simulink model "T4_ongrid_updatesolar"  (R2022b)
settings: Solver=FixedStepAuto  StartTime=0.0  StopTime=24  FixedStep=0.01  RelTol=1e-3
undefined symbols (not defined in the file): High, Low, Ts
libraries: fl_lib x142, nesl_utility x59, simulink x15, ee_lib x8, batteryecm_lib x1
(part 2 of 3)

== system T4_ongrid_updatesolar/Household8 ==
  Current Sensor : fl_lib/Electrical/Electrical Sensors/Current Sensor
  PS Divide : fl_lib/Physical Signals/Functions/PS Divide
  PS Product : fl_lib/Physical Signals/Functions/PS Product
  PS-Simulink Converter : nesl_utility/PS-Simulink Converter  PhysicalDomain=network_engine_domain  SubClassName=ps_output  LeftPortType=input  RightPortType=output  PseudoPeriodic=off  Frequencies=[]  VectorFormat=inherit  Unit=inherit  AffineConversion=off
  PS-Simulink Converter1 : nesl_utility/PS-Simulink Converter  PhysicalDomain=network_engine_domain  SubClassName=ps_output  LeftPortType=input  RightPortType=output  PseudoPeriodic=off  Frequencies=[]  VectorFormat=inherit  Unit=inherit  AffineConversion=off
  Product : Product
  "Residential power " : simulink/Sources/Repeating Sequence Interpolated  OutValues=[2.8 2.5 2 2 2.2 2.5 2.8 3.4 3.6 3.8 4 4 4 4 4 4 4 4 4 4 3.8 3.5 3.2 3]*1000  TimeValues=[0 1 2 3 4 5 6 7 8 9 10 11 12 13 14 15 16 17 18 19 20 21 22 23]  LookUpMeth=Interpolation-Use End Values  tsamp=0.01  OutMin=[]  OutMax=[]  OutDataTypeStr=double  OutputDataTypeScalingMode=double  OutDataType=fixdt(0,8)  OutScaling=2^-10
  Simscape Bus1 : SimscapeBus  HierarchyStrings=High;Low
  Simulink-PS Converter1 : nesl_utility/Simulink-PS Converter  PhysicalDomain=network_engine_domain  SubClassName=ps_input  LeftPortType=input  RightPortType=output  PseudoPeriodic=off  Frequencies=[]  NoiseDistribution=none  NoiseParameters=[]  Unit=V*A  AffineConversion=off  FilteringAndDerivatives=provide  SimscapeFilterOrder=1  InputFilterTimeConstant=0.001  UdotUserProvided=0
  Terminator : Terminator
  Variable Resistor : fl_lib/Electrical/Electrical Elements/Variable Resistor  Rmin=0 Ohm  i_specify=off  i_priority=None  i=0 A  i_nominal_specify=off  i_nominal_unit=A  i_nominal_value=1  v_specify=off  v_priority=None  v=0 V  v_nominal_specify=off  v_nominal_unit=V  v_nominal_value=1
  Vnom : fl_lib/Physical Signals/Sources/PS Constant  constant=48 V
  Voltage Sensor : fl_lib/Electrical/Electrical Sensors/Voltage Sensor
  IndustrialOut : PMIOPort  Side=Right
  wires:
  Product/1 -> Terminator/1  "power"
  PS-Simulink Converter1/1 -> Product/1  "current"
  PS-Simulink Converter/1 -> Product/2  "voltage"
  "Residential power "/1 -> Simulink-PS Converter1/1  "electrical"
  connections:
  Current Sensor/RConn1 -- PS-Simulink Converter1/LConn1
  Current Sensor/LConn1 -- Simscape Bus1/LConn1
  Voltage Sensor/RConn1 -- PS-Simulink Converter/LConn1
  Current Sensor/RConn2 -- Variable Resistor/LConn2 -- Voltage Sensor/LConn1
  IndustrialOut/RConn1 -- Simscape Bus1/RConn1
  Voltage Sensor/RConn2 -- Simscape Bus1/LConn2 -- Variable Resistor/RConn1
  Vnom/RConn1 -- PS Product/LConn2 -- PS Product/LConn1
  PS Divide/LConn2 -- Simulink-PS Converter1/RConn1
  Variable Resistor/LConn1 -- PS Divide/RConn1
  PS Divide/LConn1 -- PS Product/RConn1

== system T4_ongrid_updatesolar/Household9 ==
  Current Sensor : fl_lib/Electrical/Electrical Sensors/Current Sensor
  PS Divide : fl_lib/Physical Signals/Functions/PS Divide
  PS Product : fl_lib/Physical Signals/Functions/PS Product
  PS-Simulink Converter : nesl_utility/PS-Simulink Converter  PhysicalDomain=network_engine_domain  SubClassName=ps_output  LeftPortType=input  RightPortType=output  PseudoPeriodic=off  Frequencies=[]  VectorFormat=inherit  Unit=inherit  AffineConversion=off
  PS-Simulink Converter1 : nesl_utility/PS-Simulink Converter  PhysicalDomain=network_engine_domain  SubClassName=ps_output  LeftPortType=input  RightPortType=output  PseudoPeriodic=off  Frequencies=[]  VectorFormat=inherit  Unit=inherit  AffineConversion=off
  Product : Product
  "Residential power " : simulink/Sources/Repeating Sequence Interpolated  OutValues=[2.8 2.5 2 2 2.2 2.5 2.8 3.4 3.6 3.8 4 4 4 4 4 4 4 4 4 4 3.8 3.5 3.2 3]*1000  TimeValues=[0 1 2 3 4 5 6 7 8 9 10 11 12 13 14 15 16 17 18 19 20 21 22 23]  LookUpMeth=Interpolation-Use End Values  tsamp=0.01  OutMin=[]  OutMax=[]  OutDataTypeStr=double  OutputDataTypeScalingMode=double  OutDataType=fixdt(0,8)  OutScaling=2^-10
  Simscape Bus1 : SimscapeBus  HierarchyStrings=High;Low
  Simulink-PS Converter1 : nesl_utility/Simulink-PS Converter  PhysicalDomain=network_engine_domain  SubClassName=ps_input  LeftPortType=input  RightPortType=output  PseudoPeriodic=off  Frequencies=[]  NoiseDistribution=none  NoiseParameters=[]  Unit=V*A  AffineConversion=off  FilteringAndDerivatives=provide  SimscapeFilterOrder=1  InputFilterTimeConstant=0.001  UdotUserProvided=0
  Terminator : Terminator
  Variable Resistor : fl_lib/Electrical/Electrical Elements/Variable Resistor  Rmin=0 Ohm  i_specify=off  i_priority=None  i=0 A  i_nominal_specify=off  i_nominal_unit=A  i_nominal_value=1  v_specify=off  v_priority=None  v=0 V  v_nominal_specify=off  v_nominal_unit=V  v_nominal_value=1
  Vnom : fl_lib/Physical Signals/Sources/PS Constant  constant=48 V
  Voltage Sensor : fl_lib/Electrical/Electrical Sensors/Voltage Sensor
  IndustrialOut : PMIOPort  Side=Right
  wires:
  Product/1 -> Terminator/1  "power"
  PS-Simulink Converter1/1 -> Product/1  "current"
  PS-Simulink Converter/1 -> Product/2  "voltage"
  "Residential power "/1 -> Simulink-PS Converter1/1  "electrical"
  connections:
  Current Sensor/RConn1 -- PS-Simulink Converter1/LConn1
  Current Sensor/LConn1 -- Simscape Bus1/LConn1
  Voltage Sensor/RConn1 -- PS-Simulink Converter/LConn1
  Current Sensor/RConn2 -- Variable Resistor/LConn2 -- Voltage Sensor/LConn1
  IndustrialOut/RConn1 -- Simscape Bus1/RConn1
  Voltage Sensor/RConn2 -- Simscape Bus1/LConn2 -- Variable Resistor/RConn1
  Vnom/RConn1 -- PS Product/LConn2 -- PS Product/LConn1
  PS Divide/LConn2 -- Simulink-PS Converter1/RConn1
  Variable Resistor/LConn1 -- PS Divide/RConn1
  PS Divide/LConn1 -- PS Product/RConn1

== system T4_ongrid_updatesolar/Line1 ==
  Resistor : fl_lib/Electrical/Electrical Elements/Resistor  R=rho*l/A Ohm  i_specify=off  i_priority=None  i=0 A  i_nominal_specify=off  i_nominal_unit=A  i_nominal_value=1  v_specify=off  v_priority=None  v=0 V  v_nominal_specify=off  v_nominal_unit=V  v_nominal_value=1
  Resistor1 : fl_lib/Electrical/Electrical Elements/Resistor  R=rho*l/A Ohm  i_specify=off  i_priority=None  i=0 A  i_nominal_specify=off  i_nominal_unit=A  i_nominal_value=1  v_specify=off  v_priority=None  v=0 V  v_nominal_specify=off  v_nominal_unit=V  v_nominal_value=1
  Simscape Bus2 : SimscapeBus  HierarchyStrings=High;Low
  Simscape Bus3 : SimscapeBus  HierarchyStrings=High;Low
  In : PMIOPort  Side=Left
  Out : PMIOPort  Port=2  Side=Right
  connections:
  Simscape Bus2/LConn1 -- Resistor/LConn1
  Simscape Bus3/LConn2 -- Resistor1/RConn1
  Simscape Bus2/RConn1 -- In/RConn1
  Simscape Bus3/LConn1 -- Resistor/RConn1
  Resistor1/LConn1 -- Simscape Bus2/LConn2
  Simscape Bus3/RConn1 -- Out/RConn1

== system T4_ongrid_updatesolar/Line10 ==
  Resistor : fl_lib/Electrical/Electrical Elements/Resistor  R=rho*l/A Ohm  i_specify=off  i_priority=None  i=0 A  i_nominal_specify=off  i_nominal_unit=A  i_nominal_value=1  v_specify=off  v_priority=None  v=0 V  v_nominal_specify=off  v_nominal_unit=V  v_nominal_value=1
  Resistor1 : fl_lib/Electrical/Electrical Elements/Resistor  R=rho*l/A Ohm  i_specify=off  i_priority=None  i=0 A  i_nominal_specify=off  i_nominal_unit=A  i_nominal_value=1  v_specify=off  v_priority=None  v=0 V  v_nominal_specify=off  v_nominal_unit=V  v_nominal_value=1
  Simscape Bus2 : SimscapeBus  HierarchyStrings=High;Low
  Simscape Bus3 : SimscapeBus  HierarchyStrings=High;Low
  In : PMIOPort  Side=Left
  Out : PMIOPort  Port=2  Side=Right
  connections:
  Simscape Bus2/LConn1 -- Resistor/LConn1
  Simscape Bus3/LConn2 -- Resistor1/RConn1
  Simscape Bus2/RConn1 -- In/RConn1
  Simscape Bus3/LConn1 -- Resistor/RConn1
  Resistor1/LConn1 -- Simscape Bus2/LConn2
  Simscape Bus3/RConn1 -- Out/RConn1

== system T4_ongrid_updatesolar/Line11 ==
  Resistor : fl_lib/Electrical/Electrical Elements/Resistor  R=rho*l/A Ohm  i_specify=off  i_priority=None  i=0 A  i_nominal_specify=off  i_nominal_unit=A  i_nominal_value=1  v_specify=off  v_priority=None  v=0 V  v_nominal_specify=off  v_nominal_unit=V  v_nominal_value=1
  Resistor1 : fl_lib/Electrical/Electrical Elements/Resistor  R=rho*l/A Ohm  i_specify=off  i_priority=None  i=0 A  i_nominal_specify=off  i_nominal_unit=A  i_nominal_value=1  v_specify=off  v_priority=None  v=0 V  v_nominal_specify=off  v_nominal_unit=V  v_nominal_value=1
  Simscape Bus2 : SimscapeBus  HierarchyStrings=High;Low
  Simscape Bus3 : SimscapeBus  HierarchyStrings=High;Low
  In : PMIOPort  Side=Left
  Out : PMIOPort  Port=2  Side=Right
  connections:
  Simscape Bus3/RConn1 -- Out/RConn1
  Resistor1/LConn1 -- Simscape Bus2/LConn2
  Simscape Bus3/LConn1 -- Resistor/RConn1
  Simscape Bus2/RConn1 -- In/RConn1
  Simscape Bus3/LConn2 -- Resistor1/RConn1
  Simscape Bus2/LConn1 -- Resistor/LConn1

== system T4_ongrid_updatesolar/Line12 ==
  Resistor : fl_lib/Electrical/Electrical Elements/Resistor  R=rho*l/A Ohm  i_specify=off  i_priority=None  i=0 A  i_nominal_specify=off  i_nominal_unit=A  i_nominal_value=1  v_specify=off  v_priority=None  v=0 V  v_nominal_specify=off  v_nominal_unit=V  v_nominal_value=1
  Resistor1 : fl_lib/Electrical/Electrical Elements/Resistor  R=rho*l/A Ohm  i_specify=off  i_priority=None  i=0 A  i_nominal_specify=off  i_nominal_unit=A  i_nominal_value=1  v_specify=off  v_priority=None  v=0 V  v_nominal_specify=off  v_nominal_unit=V  v_nominal_value=1
  Simscape Bus2 : SimscapeBus  HierarchyStrings=High;Low
  Simscape Bus3 : SimscapeBus  HierarchyStrings=High;Low
  In : PMIOPort  Side=Left
  Out : PMIOPort  Port=2  Side=Right
  connections:
  Simscape Bus3/RConn1 -- Out/RConn1
  Resistor1/LConn1 -- Simscape Bus2/LConn2
  Simscape Bus3/LConn1 -- Resistor/RConn1
  Simscape Bus2/RConn1 -- In/RConn1
  Simscape Bus3/LConn2 -- Resistor1/RConn1
  Simscape Bus2/LConn1 -- Resistor/LConn1

== system T4_ongrid_updatesolar/Line13 ==
  Resistor : fl_lib/Electrical/Electrical Elements/Resistor  R=rho*l/A Ohm  i_specify=off  i_priority=None  i=0 A  i_nominal_specify=off  i_nominal_unit=A  i_nominal_value=1  v_specify=off  v_priority=None  v=0 V  v_nominal_specify=off  v_nominal_unit=V  v_nominal_value=1
  Resistor1 : fl_lib/Electrical/Electrical Elements/Resistor  R=rho*l/A Ohm  i_specify=off  i_priority=None  i=0 A  i_nominal_specify=off  i_nominal_unit=A  i_nominal_value=1  v_specify=off  v_priority=None  v=0 V  v_nominal_specify=off  v_nominal_unit=V  v_nominal_value=1
  Simscape Bus2 : SimscapeBus  HierarchyStrings=High;Low
  Simscape Bus3 : SimscapeBus  HierarchyStrings=High;Low
  In : PMIOPort  Side=Left
  Out : PMIOPort  Port=2  Side=Right
  connections:
  Simscape Bus2/LConn1 -- Resistor/LConn1
  Simscape Bus3/LConn2 -- Resistor1/RConn1
  Simscape Bus2/RConn1 -- In/RConn1
  Simscape Bus3/LConn1 -- Resistor/RConn1
  Resistor1/LConn1 -- Simscape Bus2/LConn2
  Simscape Bus3/RConn1 -- Out/RConn1

== system T4_ongrid_updatesolar/Line14 ==
  Resistor : fl_lib/Electrical/Electrical Elements/Resistor  R=rho*l/A Ohm  i_specify=off  i_priority=None  i=0 A  i_nominal_specify=off  i_nominal_unit=A  i_nominal_value=1  v_specify=off  v_priority=None  v=0 V  v_nominal_specify=off  v_nominal_unit=V  v_nominal_value=1
  Resistor1 : fl_lib/Electrical/Electrical Elements/Resistor  R=rho*l/A Ohm  i_specify=off  i_priority=None  i=0 A  i_nominal_specify=off  i_nominal_unit=A  i_nominal_value=1  v_specify=off  v_priority=None  v=0 V  v_nominal_specify=off  v_nominal_unit=V  v_nominal_value=1
  Simscape Bus2 : SimscapeBus  HierarchyStrings=High;Low
  Simscape Bus3 : SimscapeBus  HierarchyStrings=High;Low
  In : PMIOPort  Side=Left
  Out : PMIOPort  Port=2  Side=Right
  connections:
  Simscape Bus3/RConn1 -- Out/RConn1
  Resistor1/LConn1 -- Simscape Bus2/LConn2
  Simscape Bus3/LConn1 -- Resistor/RConn1
  Simscape Bus2/RConn1 -- In/RConn1
  Simscape Bus3/LConn2 -- Resistor1/RConn1
  Simscape Bus2/LConn1 -- Resistor/LConn1

== system T4_ongrid_updatesolar/Line15 ==
  Resistor : fl_lib/Electrical/Electrical Elements/Resistor  R=rho*l/A Ohm  i_specify=off  i_priority=None  i=0 A  i_nominal_specify=off  i_nominal_unit=A  i_nominal_value=1  v_specify=off  v_priority=None  v=0 V  v_nominal_specify=off  v_nominal_unit=V  v_nominal_value=1
  Resistor1 : fl_lib/Electrical/Electrical Elements/Resistor  R=rho*l/A Ohm  i_specify=off  i_priority=None  i=0 A  i_nominal_specify=off  i_nominal_unit=A  i_nominal_value=1  v_specify=off  v_priority=None  v=0 V  v_nominal_specify=off  v_nominal_unit=V  v_nominal_value=1
  Simscape Bus2 : SimscapeBus  HierarchyStrings=High;Low
  Simscape Bus3 : SimscapeBus  HierarchyStrings=High;Low
  In : PMIOPort  Side=Left
  Out : PMIOPort  Port=2  Side=Right
  connections:
  Simscape Bus2/LConn1 -- Resistor/LConn1
  Simscape Bus3/LConn2 -- Resistor1/RConn1
  Simscape Bus2/RConn1 -- In/RConn1
  Simscape Bus3/LConn1 -- Resistor/RConn1
  Resistor1/LConn1 -- Simscape Bus2/LConn2
  Simscape Bus3/RConn1 -- Out/RConn1

== system T4_ongrid_updatesolar/Line16 ==
  Resistor : fl_lib/Electrical/Electrical Elements/Resistor  R=rho*l/A Ohm  i_specify=off  i_priority=None  i=0 A  i_nominal_specify=off  i_nominal_unit=A  i_nominal_value=1  v_specify=off  v_priority=None  v=0 V  v_nominal_specify=off  v_nominal_unit=V  v_nominal_value=1
  Resistor1 : fl_lib/Electrical/Electrical Elements/Resistor  R=rho*l/A Ohm  i_specify=off  i_priority=None  i=0 A  i_nominal_specify=off  i_nominal_unit=A  i_nominal_value=1  v_specify=off  v_priority=None  v=0 V  v_nominal_specify=off  v_nominal_unit=V  v_nominal_value=1
  Simscape Bus2 : SimscapeBus  HierarchyStrings=High;Low
  Simscape Bus3 : SimscapeBus  HierarchyStrings=High;Low
  In : PMIOPort  Side=Left
  Out : PMIOPort  Port=2  Side=Right
  connections:
  Simscape Bus2/LConn1 -- Resistor/LConn1
  Simscape Bus3/LConn2 -- Resistor1/RConn1
  Simscape Bus2/RConn1 -- In/RConn1
  Simscape Bus3/LConn1 -- Resistor/RConn1
  Resistor1/LConn1 -- Simscape Bus2/LConn2
  Simscape Bus3/RConn1 -- Out/RConn1

== system T4_ongrid_updatesolar/Line17 ==
  Resistor : fl_lib/Electrical/Electrical Elements/Resistor  R=rho*l/A Ohm  i_specify=off  i_priority=None  i=0 A  i_nominal_specify=off  i_nominal_unit=A  i_nominal_value=1  v_specify=off  v_priority=None  v=0 V  v_nominal_specify=off  v_nominal_unit=V  v_nominal_value=1
  Resistor1 : fl_lib/Electrical/Electrical Elements/Resistor  R=rho*l/A Ohm  i_specify=off  i_priority=None  i=0 A  i_nominal_specify=off  i_nominal_unit=A  i_nominal_value=1  v_specify=off  v_priority=None  v=0 V  v_nominal_specify=off  v_nominal_unit=V  v_nominal_value=1
  Simscape Bus2 : SimscapeBus  HierarchyStrings=High;Low
  Simscape Bus3 : SimscapeBus  HierarchyStrings=High;Low
  In : PMIOPort  Side=Left
  Out : PMIOPort  Port=2  Side=Right
  connections:
  Simscape Bus3/RConn1 -- Out/RConn1
  Resistor1/LConn1 -- Simscape Bus2/LConn2
  Simscape Bus3/LConn1 -- Resistor/RConn1
  Simscape Bus2/RConn1 -- In/RConn1
  Simscape Bus3/LConn2 -- Resistor1/RConn1
  Simscape Bus2/LConn1 -- Resistor/LConn1

== system T4_ongrid_updatesolar/Line18 ==
  Resistor : fl_lib/Electrical/Electrical Elements/Resistor  R=rho*l/A Ohm  i_specify=off  i_priority=None  i=0 A  i_nominal_specify=off  i_nominal_unit=A  i_nominal_value=1  v_specify=off  v_priority=None  v=0 V  v_nominal_specify=off  v_nominal_unit=V  v_nominal_value=1
  Resistor1 : fl_lib/Electrical/Electrical Elements/Resistor  R=rho*l/A Ohm  i_specify=off  i_priority=None  i=0 A  i_nominal_specify=off  i_nominal_unit=A  i_nominal_value=1  v_specify=off  v_priority=None  v=0 V  v_nominal_specify=off  v_nominal_unit=V  v_nominal_value=1
  Simscape Bus2 : SimscapeBus  HierarchyStrings=High;Low
  Simscape Bus3 : SimscapeBus  HierarchyStrings=High;Low
  In : PMIOPort  Side=Left
  Out : PMIOPort  Port=2  Side=Right
  connections:
  Simscape Bus3/RConn1 -- Out/RConn1
  Resistor1/LConn1 -- Simscape Bus2/LConn2
  Simscape Bus3/LConn1 -- Resistor/RConn1
  Simscape Bus2/RConn1 -- In/RConn1
  Simscape Bus3/LConn2 -- Resistor1/RConn1
  Simscape Bus2/LConn1 -- Resistor/LConn1

== system T4_ongrid_updatesolar/Line19 ==
  Resistor : fl_lib/Electrical/Electrical Elements/Resistor  R=rho*l/A Ohm  i_specify=off  i_priority=None  i=0 A  i_nominal_specify=off  i_nominal_unit=A  i_nominal_value=1  v_specify=off  v_priority=None  v=0 V  v_nominal_specify=off  v_nominal_unit=V  v_nominal_value=1
  Resistor1 : fl_lib/Electrical/Electrical Elements/Resistor  R=rho*l/A Ohm  i_specify=off  i_priority=None  i=0 A  i_nominal_specify=off  i_nominal_unit=A  i_nominal_value=1  v_specify=off  v_priority=None  v=0 V  v_nominal_specify=off  v_nominal_unit=V  v_nominal_value=1
  Simscape Bus2 : SimscapeBus  HierarchyStrings=High;Low
  Simscape Bus3 : SimscapeBus  HierarchyStrings=High;Low
  In : PMIOPort  Side=Left
  Out : PMIOPort  Port=2  Side=Right
  connections:
  Simscape Bus2/LConn1 -- Resistor/LConn1
  Simscape Bus3/LConn2 -- Resistor1/RConn1
  Simscape Bus2/RConn1 -- In/RConn1
  Simscape Bus3/LConn1 -- Resistor/RConn1
  Resistor1/LConn1 -- Simscape Bus2/LConn2
  Simscape Bus3/RConn1 -- Out/RConn1

== system T4_ongrid_updatesolar/Line2 ==
  Resistor : fl_lib/Electrical/Electrical Elements/Resistor  R=rho*l/A Ohm  i_specify=off  i_priority=None  i=0 A  i_nominal_specify=off  i_nominal_unit=A  i_nominal_value=1  v_specify=off  v_priority=None  v=0 V  v_nominal_specify=off  v_nominal_unit=V  v_nominal_value=1
  Resistor1 : fl_lib/Electrical/Electrical Elements/Resistor  R=rho*l/A Ohm  i_specify=off  i_priority=None  i=0 A  i_nominal_specify=off  i_nominal_unit=A  i_nominal_value=1  v_specify=off  v_priority=None  v=0 V  v_nominal_specify=off  v_nominal_unit=V  v_nominal_value=1
  Simscape Bus2 : SimscapeBus  HierarchyStrings=High;Low
  Simscape Bus3 : SimscapeBus  HierarchyStrings=High;Low
  In : PMIOPort  Side=Left
  Out : PMIOPort  Port=2  Side=Right
  connections:
  Simscape Bus3/RConn1 -- Out/RConn1
  Resistor1/LConn1 -- Simscape Bus2/LConn2
  Simscape Bus3/LConn1 -- Resistor/RConn1
  Simscape Bus2/RConn1 -- In/RConn1
  Simscape Bus3/LConn2 -- Resistor1/RConn1
  Simscape Bus2/LConn1 -- Resistor/LConn1

== system T4_ongrid_updatesolar/Line20 ==
  Resistor : fl_lib/Electrical/Electrical Elements/Resistor  R=rho*l/A Ohm  i_specify=off  i_priority=None  i=0 A  i_nominal_specify=off  i_nominal_unit=A  i_nominal_value=1  v_specify=off  v_priority=None  v=0 V  v_nominal_specify=off  v_nominal_unit=V  v_nominal_value=1
  Resistor1 : fl_lib/Electrical/Electrical Elements/Resistor  R=rho*l/A Ohm  i_specify=off  i_priority=None  i=0 A  i_nominal_specify=off  i_nominal_unit=A  i_nominal_value=1  v_specify=off  v_priority=None  v=0 V  v_nominal_specify=off  v_nominal_unit=V  v_nominal_value=1
  Simscape Bus2 : SimscapeBus  HierarchyStrings=High;Low
  Simscape Bus3 : SimscapeBus  HierarchyStrings=High;Low
  In : PMIOPort  Side=Left
  Out : PMIOPort  Port=2  Side=Right
  connections:
  Simscape Bus3/RConn1 -- Out/RConn1
  Resistor1/LConn1 -- Simscape Bus2/LConn2
  Simscape Bus3/LConn1 -- Resistor/RConn1
  Simscape Bus2/RConn1 -- In/RConn1
  Simscape Bus3/LConn2 -- Resistor1/RConn1
  Simscape Bus2/LConn1 -- Resistor/LConn1

== system T4_ongrid_updatesolar/Line3 ==
  Resistor : fl_lib/Electrical/Electrical Elements/Resistor  R=rho*l/A Ohm  i_specify=off  i_priority=None  i=0 A  i_nominal_specify=off  i_nominal_unit=A  i_nominal_value=1  v_specify=off  v_priority=None  v=0 V  v_nominal_specify=off  v_nominal_unit=V  v_nominal_value=1
  Resistor1 : fl_lib/Electrical/Electrical Elements/Resistor  R=rho*l/A Ohm  i_specify=off  i_priority=None  i=0 A  i_nominal_specify=off  i_nominal_unit=A  i_nominal_value=1  v_specify=off  v_priority=None  v=0 V  v_nominal_specify=off  v_nominal_unit=V  v_nominal_value=1
  Simscape Bus2 : SimscapeBus  HierarchyStrings=High;Low
  Simscape Bus3 : SimscapeBus  HierarchyStrings=High;Low
  In : PMIOPort  Side=Left
  Out : PMIOPort  Port=2  Side=Right
  connections:
  Simscape Bus2/LConn1 -- Resistor/LConn1
  Simscape Bus3/LConn2 -- Resistor1/RConn1
  Simscape Bus2/RConn1 -- In/RConn1
  Simscape Bus3/LConn1 -- Resistor/RConn1
  Resistor1/LConn1 -- Simscape Bus2/LConn2
  Simscape Bus3/RConn1 -- Out/RConn1

== system T4_ongrid_updatesolar/Line4 ==
  Resistor : fl_lib/Electrical/Electrical Elements/Resistor  R=rho*l/A Ohm  i_specify=off  i_priority=None  i=0 A  i_nominal_specify=off  i_nominal_unit=A  i_nominal_value=1  v_specify=off  v_priority=None  v=0 V  v_nominal_specify=off  v_nominal_unit=V  v_nominal_value=1
  Resistor1 : fl_lib/Electrical/Electrical Elements/Resistor  R=rho*l/A Ohm  i_specify=off  i_priority=None  i=0 A  i_nominal_specify=off  i_nominal_unit=A  i_nominal_value=1  v_specify=off  v_priority=None  v=0 V  v_nominal_specify=off  v_nominal_unit=V  v_nominal_value=1
  Simscape Bus2 : SimscapeBus  HierarchyStrings=High;Low
  Simscape Bus3 : SimscapeBus  HierarchyStrings=High;Low
  In : PMIOPort  Side=Left
  Out : PMIOPort  Port=2  Side=Right
  connections:
  Simscape Bus3/RConn1 -- Out/RConn1
  Resistor1/LConn1 -- Simscape Bus2/LConn2
  Simscape Bus3/LConn1 -- Resistor/RConn1
  Simscape Bus2/RConn1 -- In/RConn1
  Simscape Bus3/LConn2 -- Resistor1/RConn1
  Simscape Bus2/LConn1 -- Resistor/LConn1

== system T4_ongrid_updatesolar/Line5 ==
  Resistor : fl_lib/Electrical/Electrical Elements/Resistor  R=rho*l/A Ohm  i_specify=off  i_priority=None  i=0 A  i_nominal_specify=off  i_nominal_unit=A  i_nominal_value=1  v_specify=off  v_priority=None  v=0 V  v_nominal_specify=off  v_nominal_unit=V  v_nominal_value=1
  Resistor1 : fl_lib/Electrical/Electrical Elements/Resistor  R=rho*l/A Ohm  i_specify=off  i_priority=None  i=0 A  i_nominal_specify=off  i_nominal_unit=A  i_nominal_value=1  v_specify=off  v_priority=None  v=0 V  v_nominal_specify=off  v_nominal_unit=V  v_nominal_value=1
  Simscape Bus2 : SimscapeBus  HierarchyStrings=High;Low
  Simscape Bus3 : SimscapeBus  HierarchyStrings=High;Low
  In : PMIOPort  Side=Left
  Out : PMIOPort  Port=2  Side=Right
  connections:
  Simscape Bus2/LConn1 -- Resistor/LConn1
  Simscape Bus3/LConn2 -- Resistor1/RConn1
  Simscape Bus2/RConn1 -- In/RConn1
  Simscape Bus3/LConn1 -- Resistor/RConn1
  Resistor1/LConn1 -- Simscape Bus2/LConn2
  Simscape Bus3/RConn1 -- Out/RConn1

== system T4_ongrid_updatesolar/Line6 ==
  Resistor : fl_lib/Electrical/Electrical Elements/Resistor  R=rho*l/A Ohm  i_specify=off  i_priority=None  i=0 A  i_nominal_specify=off  i_nominal_unit=A  i_nominal_value=1  v_specify=off  v_priority=None  v=0 V  v_nominal_specify=off  v_nominal_unit=V  v_nominal_value=1
  Resistor1 : fl_lib/Electrical/Electrical Elements/Resistor  R=rho*l/A Ohm  i_specify=off  i_priority=None  i=0 A  i_nominal_specify=off  i_nominal_unit=A  i_nominal_value=1  v_specify=off  v_priority=None  v=0 V  v_nominal_specify=off  v_nominal_unit=V  v_nominal_value=1
  Simscape Bus2 : SimscapeBus  HierarchyStrings=High;Low
  Simscape Bus3 : SimscapeBus  HierarchyStrings=High;Low
  In : PMIOPort  Side=Left
  Out : PMIOPort  Port=2  Side=Right
  connections:
  Simscape Bus3/RConn1 -- Out/RConn1
  Resistor1/LConn1 -- Simscape Bus2/LConn2
  Simscape Bus3/LConn1 -- Resistor/RConn1
  Simscape Bus2/RConn1 -- In/RConn1
  Simscape Bus3/LConn2 -- Resistor1/RConn1
  Simscape Bus2/LConn1 -- Resistor/LConn1

== system T4_ongrid_updatesolar/Line7 ==
  Resistor : fl_lib/Electrical/Electrical Elements/Resistor  R=rho*l/A Ohm  i_specify=off  i_priority=None  i=0 A  i_nominal_specify=off  i_nominal_unit=A  i_nominal_value=1  v_specify=off  v_priority=None  v=0 V  v_nominal_specify=off  v_nominal_unit=V  v_nominal_value=1
  Resistor1 : fl_lib/Electrical/Electrical Elements/Resistor  R=rho*l/A Ohm  i_specify=off  i_priority=None  i=0 A  i_nominal_specify=off  i_nominal_unit=A  i_nominal_value=1  v_specify=off  v_priority=None  v=0 V  v_nominal_specify=off  v_nominal_unit=V  v_nominal_value=1
  Simscape Bus2 : SimscapeBus  HierarchyStrings=High;Low
  Simscape Bus3 : SimscapeBus  HierarchyStrings=High;Low
  In : PMIOPort  Side=Left
  Out : PMIOPort  Port=2  Side=Right
  connections:
  Simscape Bus2/LConn1 -- Resistor/LConn1
  Simscape Bus3/LConn2 -- Resistor1/RConn1
  Simscape Bus2/RConn1 -- In/RConn1
  Simscape Bus3/LConn1 -- Resistor/RConn1
  Resistor1/LConn1 -- Simscape Bus2/LConn2
  Simscape Bus3/RConn1 -- Out/RConn1

== system T4_ongrid_updatesolar/Line8 ==
  Resistor : fl_lib/Electrical/Electrical Elements/Resistor  R=rho*l/A Ohm  i_specify=off  i_priority=None  i=0 A  i_nominal_specify=off  i_nominal_unit=A  i_nominal_value=1  v_specify=off  v_priority=None  v=0 V  v_nominal_specify=off  v_nominal_unit=V  v_nominal_value=1
  Resistor1 : fl_lib/Electrical/Electrical Elements/Resistor  R=rho*l/A Ohm  i_specify=off  i_priority=None  i=0 A  i_nominal_specify=off  i_nominal_unit=A  i_nominal_value=1  v_specify=off  v_priority=None  v=0 V  v_nominal_specify=off  v_nominal_unit=V  v_nominal_value=1
  Simscape Bus2 : SimscapeBus  HierarchyStrings=High;Low
  Simscape Bus3 : SimscapeBus  HierarchyStrings=High;Low
  In : PMIOPort  Side=Left
  Out : PMIOPort  Port=2  Side=Right
  connections:
  Simscape Bus2/LConn1 -- Resistor/LConn1
  Simscape Bus3/LConn2 -- Resistor1/RConn1
  Simscape Bus2/RConn1 -- In/RConn1
  Simscape Bus3/LConn1 -- Resistor/RConn1
  Resistor1/LConn1 -- Simscape Bus2/LConn2
  Simscape Bus3/RConn1 -- Out/RConn1

== system T4_ongrid_updatesolar/Line9 ==
  Resistor : fl_lib/Electrical/Electrical Elements/Resistor  R=rho*l/A Ohm  i_specify=off  i_priority=None  i=0 A  i_nominal_specify=off  i_nominal_unit=A  i_nominal_value=1  v_specify=off  v_priority=None  v=0 V  v_nominal_specify=off  v_nominal_unit=V  v_nominal_value=1
  Resistor1 : fl_lib/Electrical/Electrical Elements/Resistor  R=rho*l/A Ohm  i_specify=off  i_priority=None  i=0 A  i_nominal_specify=off  i_nominal_unit=A  i_nominal_value=1  v_specify=off  v_priority=None  v=0 V  v_nominal_specify=off  v_nominal_unit=V  v_nominal_value=1
  Simscape Bus2 : SimscapeBus  HierarchyStrings=High;Low
  Simscape Bus3 : SimscapeBus  HierarchyStrings=High;Low
  In : PMIOPort  Side=Left
  Out : PMIOPort  Port=2  Side=Right
  connections:
  Simscape Bus3/RConn1 -- Out/RConn1
  Resistor1/LConn1 -- Simscape Bus2/LConn2
  Simscape Bus3/LConn1 -- Resistor/RConn1
  Simscape Bus2/RConn1 -- In/RConn1
  Simscape Bus3/LConn2 -- Resistor1/RConn1
  Simscape Bus2/LConn1 -- Resistor/LConn1

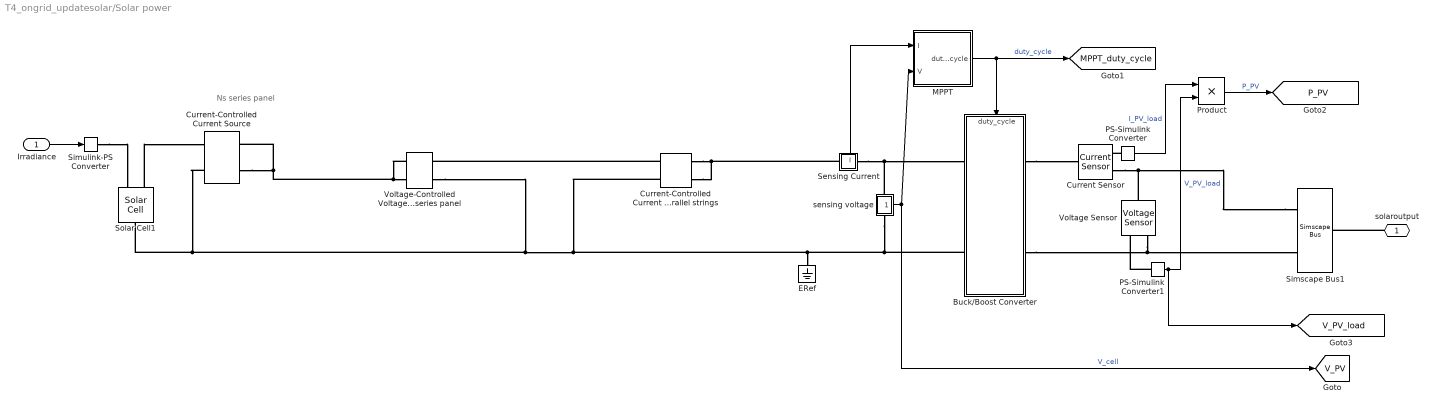
== system T4_ongrid_updatesolar/Solar power ==
  note: Ns series panel
  Irradiance : Inport
  Buck/Boost Converter : Subsystem
      settings: PortSchema="{\"entries\":[{\"content\":{\"sides\":[{\"content\":{\"connectorIds\":[\"LConn1\",\"LConn2\"]},\"type\":\"ConnectorPlacement.EquallySpacedRectSide\",\"uuid\":\"5c021c6f-6d43-4834-8d7d-5513bb4d55a2\"},{\"content\":{\"connectorIds\":[\"RConn1\",\"RConn2\"],\"side\":\"RIGHT\"},\"type\":\"ConnectorPlacement.EquallySpacedRectSide\",\"uuid\":\"9a583822-2cc1-49ae-b5aa-706b08d37e90\"},{\"content\":{\"connectorIds\":[\"In1\"],\"side\":\"TOP\"},\"type\":\"ConnectorPlacement.EquallySpacedRectSide\",\"uuid\":\"d4d092e8-f797-44a8-a681-f8c20d4ba78f\"}]},\"type\":\"ConnectorPlacement.EquallySpacedConnector\",\"uuid\":\"2126b667-6bdd-4954-a062-f2cc2f0ec1c9\"}],\"packageUris\":[\"http://schema.mathworks.com/mf0/Connector/R2020b\"],\"version\":\"1.0\"}"
  Current Sensor : fl_lib/Electrical/Electrical Sensors/Current Sensor
  Current-Controlled Current Source : fl_lib/Electrical/Electrical Sources/Current-Controlled Current Source  K=-1*(9-1)  i1_specify=off  i1_priority=None  i1=0 A  i1_nominal_specify=off  i1_nominal_unit=A  i1_nominal_value=1  i2_specify=off  i2_priority=None  i2=0 A  i2_nominal_specify=off  i2_nominal_unit=A  i2_nominal_value=1
      settings: InternalSimscapePortConfiguration="{\"Bottom\":[],\"Left\":[{\"id\":\"p1\",\"label\":\"+\",\"type\":\"foundation.electrical.electrical\"},{\"id\":\"head\",\"label\":\"\",\"type\":\"foundation.electrical.electrical\"}],\"Right\":[{\"id\":\"n1\",\"label\":\"-\",\"type\":\"foundation.electrical.electrical\"},{\"id\":\"tail\",\"label\":\"\",\"type\":\"foundation.electrical.electrical\"}],\"Top\":[]}"
  Current-Controlled Current Source- Scale panel current to Np parallel strings : fl_lib/Electrical/Electrical Sources/Current-Controlled Current Source  K=-1*(10-1)  i1_specify=off  i1_priority=None  i1=0 A  i1_nominal_specify=off  i1_nominal_unit=A  i1_nominal_value=1  i2_specify=off  i2_priority=None  i2=0 A  i2_nominal_specify=off  i2_nominal_unit=A  i2_nominal_value=1
      settings: InternalSimscapePortConfiguration="{\"Bottom\":[],\"Left\":[{\"id\":\"p1\",\"label\":\"+\",\"type\":\"foundation.electrical.electrical\"},{\"id\":\"head\",\"label\":\"\",\"type\":\"foundation.electrical.electrical\"}],\"Right\":[{\"id\":\"n1\",\"label\":\"-\",\"type\":\"foundation.electrical.electrical\"},{\"id\":\"tail\",\"label\":\"\",\"type\":\"foundation.electrical.electrical\"}],\"Top\":[]}"
  ERef : fl_lib/Electrical/Electrical Elements/Electrical Reference
  MPPT : Subsystem
  PS-Simulink Converter : nesl_utility/PS-Simulink Converter  PhysicalDomain=network_engine_domain  SubClassName=ps_output  LeftPortType=input  RightPortType=output  PseudoPeriodic=off  Frequencies=[]  VectorFormat=1-D array  Unit=inherit  AffineConversion=off
  PS-Simulink Converter1 : nesl_utility/PS-Simulink Converter  PhysicalDomain=network_engine_domain  SubClassName=ps_output  LeftPortType=input  RightPortType=output  PseudoPeriodic=off  Frequencies=[]  VectorFormat=1-D array  Unit=inherit  AffineConversion=off
  Product : Product
  Sensing Current : Subsystem
      settings: PortSchema="{\"entries\":[{\"content\":{\"sides\":[{\"content\":{\"connectorIds\":[\"LConn1\"]},\"type\":\"ConnectorPlacement.EquallySpacedRectSide\",\"uuid\":\"08eaf192-3836-4d70-9f6a-c3aee0977ea6\"},{\"content\":{\"connectorIds\":[\"RConn1\"],\"side\":\"RIGHT\"},\"type\":\"ConnectorPlacement.EquallySpacedRectSide\",\"uuid\":\"69615d36-c1bf-4d31-b3e4-77c73286e7c7\"},{\"content\":{\"connectorIds\":[\"Out1\"],\"side\":\"TOP\"},\"type\":\"ConnectorPlacement.EquallySpacedRectSide\",\"uuid\":\"21e31d90-f675-47e5-98f5-1bf7e6a5fdbe\"}]},\"type\":\"ConnectorPlacement.EquallySpacedConnector\",\"uuid\":\"068abd2e-abc9-41d7-b40e-d83d3e3b9346\"}],\"packageUris\":[\"http://schema.mathworks.com/mf0/Connector/R2020b\"],\"version\":\"1.0\"}"
      mask Display: disp('i')
  Simscape Bus1 : SimscapeBus  HierarchyStrings=High;Low
  Simulink-PS Converter : nesl_utility/Simulink-PS Converter  PhysicalDomain=network_engine_domain  SubClassName=ps_input  LeftPortType=input  RightPortType=output  PseudoPeriodic=off  Frequencies=[]  NoiseDistribution=none  NoiseParameters=[]  Unit=1  AffineConversion=off  FilteringAndDerivatives=provide  SimscapeFilterOrder=1  InputFilterTimeConstant=0.001  UdotUserProvided=0
  Solar Cell1 : ee_lib/Sources/Solar Cell  Tag={'toolbox/physmod/elec/library/m/ee_lib_parts';'Sources/Solar_Cell/Amerisolar/AS_6M30_HC_320W.xml'}  prm=1  Isc=10.00 A  Voc=0.673 V  Is=3.24823447983853e-07 A  Is2=9.37081970792037e-10 A  Iph=10.140005507508 A  Ir0=1000 W/m^2  ec=1.5  N2=2.60259908345858  Rs=0 Ohm  Rp=682.95993142779 Ohm  N_series=60  N_parallel=1  TIPH1=0.000499942933005141 1/K  EG=1.12 eV  TXIS1=4.23641510120988  TXIS2=16.2689137700667  TRS1=0.243341028305912  TRP1=0 % Parameter not set  Tmeas=25 degC  TFIXED=25 degC  thermal_mass=100 % Parameter not set J/K  initial_temperature=25 degC
      settings: AttributesFormatString=Amerisolar:AS_6M30_HC_320W
  Voltage Sensor : fl_lib/Electrical/Electrical Sensors/Voltage Sensor
  Voltage-Controlled Voltage Source - Scale panel voltage to Ns series panel : fl_lib/Electrical/Electrical Sources/Voltage-Controlled Voltage Source  K=-1*(5-1)  v1_specify=off  v1_priority=None  v1=0 V  v1_nominal_specify=off  v1_nominal_unit=V  v1_nominal_value=1  v2_specify=off  v2_priority=None  v2=0 V  v2_nominal_specify=off  v2_nominal_unit=V  v2_nominal_value=1
      settings: InternalSimscapePortConfiguration="{\"Bottom\":[],\"Left\":[{\"id\":\"p1\",\"label\":\"+\",\"type\":\"foundation.electrical.electrical\"},{\"id\":\"p2\",\"label\":\"+\",\"type\":\"foundation.electrical.electrical\"}],\"Right\":[{\"id\":\"n1\",\"label\":\"-\",\"type\":\"foundation.electrical.electrical\"},{\"id\":\"n2\",\"label\":\"-\",\"type\":\"foundation.electrical.electrical\"}],\"Top\":[]}"
  sensing voltage : Subsystem
      settings: PortSchema="{\"entries\":[{\"content\":{\"sides\":[{\"content\":{\"connectorIds\":[\"LConn1\"]},\"type\":\"ConnectorPlacement.EquallySpacedRectSide\",\"uuid\":\"08eaf192-3836-4d70-9f6a-c3aee0977ea6\"},{\"content\":{\"connectorIds\":[\"RConn1\"],\"side\":\"RIGHT\"},\"type\":\"ConnectorPlacement.EquallySpacedRectSide\",\"uuid\":\"69615d36-c1bf-4d31-b3e4-77c73286e7c7\"},{\"content\":{\"connectorIds\":[],\"side\":\"TOP\"},\"type\":\"ConnectorPlacement.EquallySpacedRectSide\",\"uuid\":\"21e31d90-f675-47e5-98f5-1bf7e6a5fdbe\"},{\"content\":{\"connectorIds\":[\"Out1\"],\"side\":\"BOTTOM\"},\"type\":\"ConnectorPlacement.EquallySpacedRectSide\",\"uuid\":\"23a77980-6beb-4147-b48e-adf9e1983263\"}]},\"type\":\"ConnectorPlacement.EquallySpacedConnector\",\"uuid\":\"068abd2e-abc9-41d7-b40e-d83d3e3b9346\"}],\"packageUris\":[\"http://schema.mathworks.com/mf0/Connector/R2020b\"],\"version\":\"1.0\"}"
      mask Display: disp('v')
  solaroutput : PMIOPort  Side=Left
  tag scope: MPPT_duty_cycle=global, P_PV=global, V_PV=global, V_PV_load=global
  wires:
  PS-Simulink Converter1/1 -> [V_PV_load], Product/2  "V_PV_load"
  MPPT/1(duty_cycle) -> [MPPT_duty_cycle], Buck/Boost Converter/1(duty_cycle)  "duty_cycle"
  Sensing Current/1(I) -> MPPT/1(I)
  PS-Simulink Converter/1 -> Product/1  "I_PV_load"
  sensing voltage/1(V) -> [V_PV], MPPT/2(V)  "V_cell"
  Product/1 -> [P_PV]  "P_PV"
  Irradiance/1 -> Simulink-PS Converter/1
  connections:
  Buck/Boost Converter/RConn2 -- Voltage Sensor/RConn2 -- Simscape Bus1/LConn2
  Simscape Bus1/LConn1 -- Voltage Sensor/LConn1 -- Current Sensor/RConn2
  sensing voltage/LConn1 -- Sensing Current/RConn1 -- Buck/Boost Converter/LConn1
  solaroutput/RConn1 -- Simscape Bus1/RConn1
  Buck/Boost Converter/RConn1 -- Current Sensor/LConn1
  PS-Simulink Converter/LConn1 -- Current Sensor/RConn1
  PS-Simulink Converter1/LConn1 -- Voltage Sensor/RConn1
  Current-Controlled Current Source/RConn2 -- Voltage-Controlled Voltage Source - Scale panel voltage to Ns series panel/RConn1 -- Voltage-Controlled Voltage Source - Scale panel voltage to Ns series panel/RConn2 -- Current-Controlled Current Source/RConn1
  Buck/Boost Converter/LConn2 -- sensing voltage/RConn1 -- Current-Controlled Current Source- Scale panel current to Np parallel strings/LConn2 -- Voltage-Controlled Voltage Source - Scale panel voltage to Ns series panel/LConn1 -- Current-Controlled Current Source/LConn2 -- Solar Cell1/RConn1 -- ERef/LConn1
  Current-Controlled Current Source- Scale panel current to Np parallel strings/RConn1 -- Sensing Current/LConn1 -- Current-Controlled Current Source- Scale panel current to Np parallel strings/RConn2
  Simulink-PS Converter/RConn1 -- Solar Cell1/LConn1
  Solar Cell1/LConn2 -- Current-Controlled Current Source/LConn1
  Current-Controlled Current Source- Scale panel current to Np parallel strings/LConn1 -- Voltage-Controlled Voltage Source - Scale panel voltage to Ns series panel/LConn2

== system T4_ongrid_updatesolar/Subsystem ==
  Scope : Scope  NumInputPorts=3
  Scope1 : Scope  NumInputPorts=3
  Scope2 : Scope
  wires:
  [P_PV] -> Scope/1
  [V_PV_load] -> Scope/3
  [V_PV] -> Scope/2
  [Residential_power1] -> Scope1/1
  [P_WIND] -> Scope2/1

== system T4_ongrid_updatesolar/Subsystem10 ==
  Resistor : fl_lib/Electrical/Electrical Elements/Resistor  R=rho*l/A Ohm  i_specify=off  i_priority=None  i=0 A  i_nominal_specify=off  i_nominal_unit=A  i_nominal_value=1  v_specify=off  v_priority=None  v=0 V  v_nominal_specify=off  v_nominal_unit=V  v_nominal_value=1
  Resistor1 : fl_lib/Electrical/Electrical Elements/Resistor  R=rho*l/A Ohm  i_specify=off  i_priority=None  i=0 A  i_nominal_specify=off  i_nominal_unit=A  i_nominal_value=1  v_specify=off  v_priority=None  v=0 V  v_nominal_specify=off  v_nominal_unit=V  v_nominal_value=1
  Simscape Bus2 : SimscapeBus  HierarchyStrings=High;Low
  Simscape Bus3 : SimscapeBus  HierarchyStrings=High;Low
  In : PMIOPort  Side=Left
  Out : PMIOPort  Port=2  Side=Right
  connections:
  Simscape Bus3/RConn1 -- Out/RConn1
  Resistor1/LConn1 -- Simscape Bus2/LConn2
  Simscape Bus3/LConn1 -- Resistor/RConn1
  Simscape Bus2/RConn1 -- In/RConn1
  Simscape Bus3/LConn2 -- Resistor1/RConn1
  Simscape Bus2/LConn1 -- Resistor/LConn1

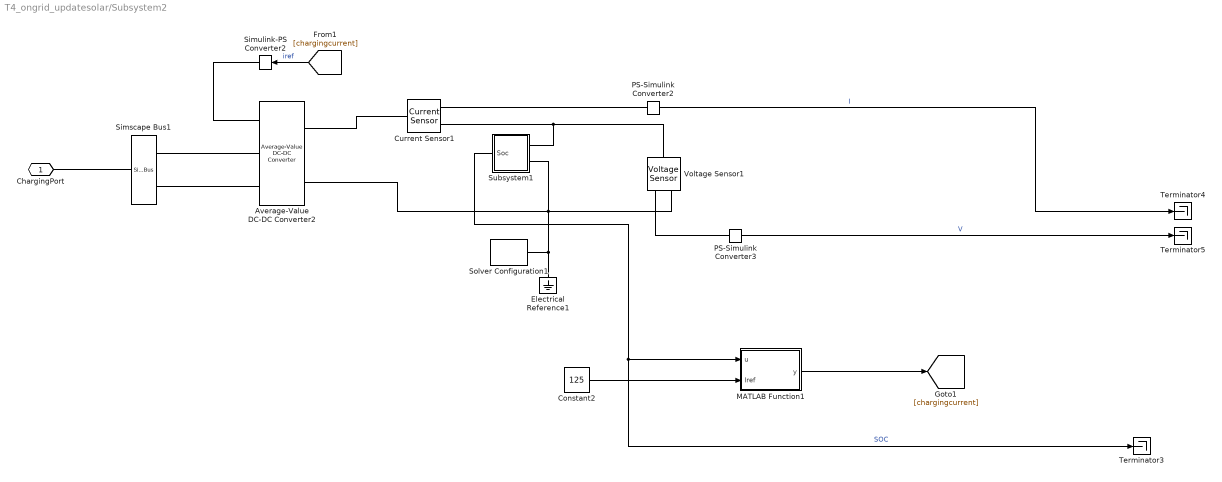
== system T4_ongrid_updatesolar/Subsystem2 ==
  Average-Value DC-DC Converter2 : ee_lib/Semiconductors & Converters/Converters/Average-Value DC-DC Converter  control_option=ee.enum.converters.controlinput.current  converter_type=ee.enum.converters.dcdctype.buckboost  efficiency_option=ee.enum.converters.efficiency.constant  efficiency_fixed=100  i_vec=[0, 2, 5] A  efficiency_vec=[90, 95, 98]
      settings: InternalSimscapePortConfiguration="{\"Bottom\":[],\"Left\":[{\"id\":\"Iref\",\"label\":\"Iref\",\"type\":\"input\"},{\"id\":\"p1\",\"label\":\"1+\",\"type\":\"foundation.electrical.electrical\"},{\"id\":\"n1\",\"label\":\"1-\",\"type\":\"foundation.electrical.electrical\"}],\"Right\":[{\"id\":\"p2\",\"label\":\"2+\",\"type\":\"foundation.electrical.electrical\"},{\"id\":\"n2\",\"label\":\"2-\",\"type\":\"foundation.electrical.electrical\"}],\"Top\":[]}"
  Constant2 : Constant  Value=125
  Current Sensor1 : fl_lib/Electrical/Electrical Sensors/Current Sensor
  Electrical Reference1 : fl_lib/Electrical/Electrical Elements/Electrical Reference
  MATLAB Function1 : MATLAB Function  TreatAsAtomicUnit=on
  PS-Simulink Converter2 : nesl_utility/PS-Simulink Converter  PhysicalDomain=network_engine_domain  SubClassName=ps_output  LeftPortType=input  RightPortType=output  PseudoPeriodic=off  Frequencies=[]  VectorFormat=inherit  Unit=inherit  AffineConversion=off
  PS-Simulink Converter3 : nesl_utility/PS-Simulink Converter  PhysicalDomain=network_engine_domain  SubClassName=ps_output  LeftPortType=input  RightPortType=output  PseudoPeriodic=off  Frequencies=[]  VectorFormat=inherit  Unit=inherit  AffineConversion=off
  Simscape Bus1 : SimscapeBus  HierarchyStrings=High;Low
  Simulink-PS Converter2 : nesl_utility/Simulink-PS Converter  PhysicalDomain=network_engine_domain  SubClassName=ps_input  LeftPortType=input  RightPortType=output  PseudoPeriodic=off  Frequencies=[]  NoiseDistribution=none  NoiseParameters=[]  Unit=1  AffineConversion=off  FilteringAndDerivatives=provide  SimscapeFilterOrder=1  InputFilterTimeConstant=0.001  UdotUserProvided=0
  Solver Configuration1 : nesl_utility/Solver Configuration  PhysicalDomain=network_engine_domain  SubClassName=solver  LeftPortType=input  RightPortType=generic  Tones=[]  Harmonics=[]  SimulateNoise=off  Profile=off  UseLocalSampling=off  EnableSwitchedLinearOptims=on  FrequencyDomain=off  UseCCode=off  RelTol=0.001  AbsTol=0.001  MinStep=1e-09  ToWorkspace=off  RevertToSquareIcSolve=off  NumHomotopyIterations=100  PhasorMode=off  PhasorModeNumHarmonics=1  ConsistencySolver=NEWTON_XTOL_AFTER_FTOL  IndexReductionMethod=DerivativeReplacement  DoDC=off  ResidualTolerance=1e-09  ConsistencyTolSource=GLOBAL  ConsistencyAbsTol=0.001  ConsistencyRelTol=0.001  ConsistencyTolFactor=0.001  UseLocalSolver=off  LocalSolverChoice=NE_BACKWARD_EULER_ADVANCER  ResolveIndetEquations=on  FunctionEvalNumThread=1  LocalSolverSampleTime=0.001  DoFixedCost=off  MaxNonlinIter=3  MaxModeIter=2  ComputeImpulses=off  ImpulseIterations=2  LinearAlgebra=auto  LinearAlgebraNumThread=0  EquationFormulation=NE_TIME_EF  DelaysMemoryBudget=1024  AutomaticFiltering=on  FilteringTimeConstant=0.001  PartitionStorageMethod=AS_NEEDED  PartitionMemoryBudget=1024  PartitionMethod=ROBUST
  Subsystem1 : Subsystem
  Terminator3 : Terminator
  Terminator4 : Terminator
  Terminator5 : Terminator
  Voltage Sensor1 : fl_lib/Electrical/Electrical Sensors/Voltage Sensor
  ChargingPort : PMIOPort  Side=Right
  wires:
  Constant2/1 -> MATLAB Function1/2(Iref)
  PS-Simulink Converter2/1 -> Terminator4/1  "I"
  Subsystem1/1(Soc) -> MATLAB Function1/1(u), Terminator3/1  "SOC"
  MATLAB Function1/1(y) -> [chargingcurrent]
  [chargingcurrent] -> Simulink-PS Converter2/1  "iref"
  PS-Simulink Converter3/1 -> Terminator5/1  "V"
  connections:
  Simscape Bus1/RConn1 -- ChargingPort/RConn1
  Average-Value DC-DC Converter2/LConn2 -- Simscape Bus1/LConn1
  Current Sensor1/LConn1 -- Average-Value DC-DC Converter2/RConn1
  Current Sensor1/RConn1 -- PS-Simulink Converter2/LConn1
  Voltage Sensor1/RConn2 -- Average-Value DC-DC Converter2/RConn2 -- Subsystem1/LConn2 -- Electrical Reference1/LConn1 -- Solver Configuration1/RConn1
  Voltage Sensor1/RConn1 -- PS-Simulink Converter3/LConn1
  Simscape Bus1/LConn2 -- Average-Value DC-DC Converter2/LConn3
  Simulink-PS Converter2/RConn1 -- Average-Value DC-DC Converter2/LConn1
  Current Sensor1/RConn2 -- Subsystem1/LConn1 -- Voltage Sensor1/LConn1

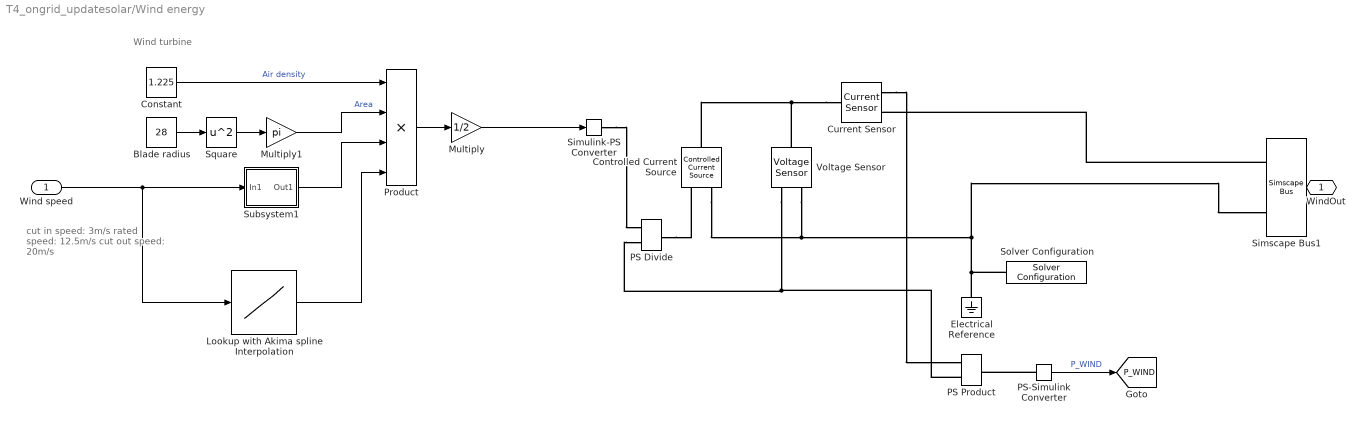
== system T4_ongrid_updatesolar/Wind energy ==
  note: cut in speed: 3m/s
      | rated speed: 12.5m/s
      | cut out speed: 20m/s
  note: Wind turbine
  Wind speed : Inport
  Blade radius : Constant  Value=28
  Constant : Constant  Value=1.225
  Controlled Current Source : fl_lib/Electrical/Electrical Sources/Controlled Current Source
  Current Sensor : fl_lib/Electrical/Electrical Sensors/Current Sensor
  Electrical Reference : fl_lib/Electrical/Electrical Elements/Electrical Reference
  Lookup with Akima spline Interpolation : Lookup_n-D  NumberOfTableDimensions=1  BreakpointsForDimension1=[0;1;2;3;4;5;6;7;8;9;10;11;12;13;14;15;16;17;18;19;20;21;22;23;24;25;26;27;28]  Table=[0;0;0;0.228;0.322;0.38;0.408;0.413;0.418;0.419;0.419;0.401;0.378;0.305;0.244;0.199;0.164;0.136;0.115;0.098;0.084;0.072;0.063;0.055;0.048;0.042;0;0;0]  InterpMethod=Akima spline  InternalRulePriority=Speed  OutDataTypeStr=double  RndMeth=Simplest
  Multiply : Gain  Gain=1/2
  Multiply1 : Gain  Gain=pi
  PS Divide : fl_lib/Physical Signals/Functions/PS Divide
  PS Product : fl_lib/Physical Signals/Functions/PS Product
  PS-Simulink Converter : nesl_utility/PS-Simulink Converter  PhysicalDomain=network_engine_domain  SubClassName=ps_output  LeftPortType=input  RightPortType=output  PseudoPeriodic=off  Frequencies=[]  VectorFormat=inherit  Unit=inherit  AffineConversion=off
  Product : Product  Inputs=4
  Simscape Bus1 : SimscapeBus  HierarchyStrings=High;Low
  Simulink-PS Converter : nesl_utility/Simulink-PS Converter  PhysicalDomain=network_engine_domain  SubClassName=ps_input  LeftPortType=input  RightPortType=output  PseudoPeriodic=off  Frequencies=[]  NoiseDistribution=none  NoiseParameters=[]  Unit=A*V  AffineConversion=off  FilteringAndDerivatives=provide  SimscapeFilterOrder=1  InputFilterTimeConstant=0.001  UdotUserProvided=0
  Solver Configuration : nesl_utility/Solver Configuration  PhysicalDomain=network_engine_domain  SubClassName=solver  LeftPortType=input  RightPortType=generic  Tones=[]  Harmonics=[]  SimulateNoise=off  Profile=off  UseLocalSampling=off  EnableSwitchedLinearOptims=on  FrequencyDomain=off  UseCCode=off  RelTol=0.001  AbsTol=0.001  MinStep=1e-09  ToWorkspace=off  RevertToSquareIcSolve=off  NumHomotopyIterations=100  PhasorMode=off  PhasorModeNumHarmonics=1  ConsistencySolver=NEWTON_XTOL_AFTER_FTOL  IndexReductionMethod=DerivativeReplacement  DoDC=off  ResidualTolerance=1e-09  ConsistencyTolSource=GLOBAL  ConsistencyAbsTol=0.001  ConsistencyRelTol=0.001  ConsistencyTolFactor=0.001  UseLocalSolver=off  LocalSolverChoice=NE_BACKWARD_EULER_ADVANCER  ResolveIndetEquations=on  FunctionEvalNumThread=1  LocalSolverSampleTime=0.001  DoFixedCost=off  MaxNonlinIter=3  MaxModeIter=2  ComputeImpulses=off  ImpulseIterations=2  LinearAlgebra=auto  LinearAlgebraNumThread=0  EquationFormulation=NE_TIME_EF  DelaysMemoryBudget=1024  AutomaticFiltering=on  FilteringTimeConstant=0.001  PartitionStorageMethod=AS_NEEDED  PartitionMemoryBudget=1024  PartitionMethod=ROBUST
  Square : Math  Operator=square
  Subsystem1 : Subsystem
      mask Display: disp('Vw^3');
  Voltage Sensor : fl_lib/Electrical/Electrical Sensors/Voltage Sensor
  WindOut : PMIOPort  Side=Right
  tag scope: P_WIND=global
  wires:
  PS-Simulink Converter/1 -> [P_WIND]  "P_WIND"
  Multiply/1 -> Simulink-PS Converter/1
  Lookup with Akima spline Interpolation/1 -> Product/4
  Multiply1/1 -> Product/2  "Area"
  Blade radius/1 -> Square/1
  Square/1 -> Multiply1/1
  Constant/1 -> Product/1  "Air density"
  Wind speed/1 -> Lookup with Akima spline Interpolation/1, Subsystem1/1(In1)
  Product/1 -> Multiply/1
  Subsystem1/1(Out1) -> Product/3
  connections:
  PS Divide/RConn1 -- Controlled Current Source/RConn1
  Voltage Sensor/RConn2 -- Controlled Current Source/RConn2 -- Electrical Reference/LConn1 -- Solver Configuration/RConn1 -- Simscape Bus1/LConn2
  Simscape Bus1/LConn1 -- Current Sensor/RConn2
  PS Divide/LConn2 -- Voltage Sensor/RConn1 -- PS Product/LConn2
  PS-Simulink Converter/LConn1 -- PS Product/RConn1
  Current Sensor/LConn1 -- Controlled Current Source/LConn1 -- Voltage Sensor/LConn1
  Current Sensor/RConn1 -- PS Product/LConn1
  Simulink-PS Converter/RConn1 -- PS Divide/LConn1
  WindOut/RConn1 -- Simscape Bus1/RConn1

== system T4_ongrid_updatesolar/Before t,off/Simscape2 ==
  Current Sensor : fl_lib/Electrical/Electrical Sensors/Current Sensor
  PS-S : nesl_utility/PS-Simulink Converter  PhysicalDomain=network_engine_domain  SubClassName=ps_output  LeftPortType=input  RightPortType=output  PseudoPeriodic=off  Frequencies=[]  VectorFormat=1-D array  Unit=A  AffineConversion=off
  + : PMIOPort  Side=Left
  - : PMIOPort  Port=2  Side=Left
  tag scope: ReplaceLine=global
  wires:
  PS-S/1 -> [ReplaceLine]  "current"
  connections:
  PS-S/LConn1 -- Current Sensor/RConn1
  Current Sensor/LConn1 -- +/RConn1
  -/RConn1 -- Current Sensor/RConn2

== system T4_ongrid_updatesolar/Solar power/Buck//Boost Converter ==
  duty_cycle : Inport
  Average-Value DC-DC Converter : ee_lib/Semiconductors & Converters/Converters/Average-Value DC-DC Converter  control_option=ee.enum.converters.controlinput.dutycycle  converter_type=ee.enum.converters.dcdctype.buckboost  efficiency_option=ee.enum.converters.efficiency.constant  efficiency_fixed=100  i_vec=[0, 2, 5] A  efficiency_vec=[90, 95, 98]
      settings: InternalSimscapePortConfiguration="{\"Bottom\":[],\"Left\":[{\"id\":\"DutyCycle\",\"label\":\"DutyCycle\",\"type\":\"input\"},{\"id\":\"p1\",\"label\":\"1+\",\"type\":\"foundation.electrical.electrical\"},{\"id\":\"n1\",\"label\":\"1-\",\"type\":\"foundation.electrical.electrical\"}],\"Right\":[{\"id\":\"p2\",\"label\":\"2+\",\"type\":\"foundation.electrical.electrical\"},{\"id\":\"n2\",\"label\":\"2-\",\"type\":\"foundation.electrical.electrical\"}],\"Top\":[]}"
  Simulink-PS Converter : nesl_utility/Simulink-PS Converter  PhysicalDomain=network_engine_domain  SubClassName=ps_input  LeftPortType=input  RightPortType=output  PseudoPeriodic=off  Frequencies=[]  NoiseDistribution=none  NoiseParameters=[]  Unit=1  AffineConversion=off  FilteringAndDerivatives=provide  SimscapeFilterOrder=1  InputFilterTimeConstant=0.001  UdotUserProvided=0
  Unit Delay : UnitDelay  InitialCondition=0.8  SampleTime=-1  HasFrameUpgradeWarning=on
  +s : PMIOPort  Side=Left
  -s : PMIOPort  Port=2  Side=Left
  -l : PMIOPort  Port=3  Side=Right
  +l : PMIOPort  Port=4  Side=Right
  wires:
  Unit Delay/1 -> Simulink-PS Converter/1
  duty_cycle/1 -> Unit Delay/1
  connections:
  Average-Value DC-DC Converter/RConn1 -- -l/RConn1
  +l/RConn1 -- Average-Value DC-DC Converter/RConn2
  Simulink-PS Converter/RConn1 -- Average-Value DC-DC Converter/LConn1
  Average-Value DC-DC Converter/LConn3 -- -s/RConn1
  +s/RConn1 -- Average-Value DC-DC Converter/LConn2

== system T4_ongrid_updatesolar/Solar power/MPPT ==
  note: Initial value for D output (Dinit)
  note: Increment value used to increase/decrease (DeltaD)
  note: Upper limit for D (Dmax)
  note: Lower limit for D (Dmin)
  I : Inport
  V : Inport  Port=2
  Enable MPPT : Step  Time=0.1  SampleTime=0.01
  Iph_ : Constant  Value=0.8
  Iph_1 : Constant  Value=0.85
  Iph_2 : Constant  Value=0.1
  Iph_3 : Constant  Value=3e-3*0.5
  "MPPT Controller using Perturb & Observe technique " : MATLAB Function  SystemSampleTime=Ts
  Mux : Mux
  Unit Delay : UnitDelay  InitialCondition=0.5  SampleTime=-1  HasFrameUpgradeWarning=on
  duty_cycle : Outport
  wires:
  V/1 -> "MPPT Controller using Perturb & Observe technique "/3(V)
  Mux/1 -> "MPPT Controller using Perturb & Observe technique "/1(Param)
  Iph_1/1 -> Mux/2
  Iph_/1 -> Mux/1
  Iph_2/1 -> Mux/3
  "MPPT Controller using Perturb & Observe technique "/1(D) -> Unit Delay/1  "duty_cycle"
  Iph_3/1 -> Mux/4
  Enable MPPT/1 -> "MPPT Controller using Perturb & Observe technique "/2(Enabled)
  I/1 -> "MPPT Controller using Perturb & Observe technique "/4(I)
  Unit Delay/1 -> duty_cycle/1

== system T4_ongrid_updatesolar/Solar power/Sensing Current ==
  Current Sensor : fl_lib/Electrical/Electrical Sensors/Current Sensor
  PS-Simulink/I : nesl_utility/PS-Simulink Converter  PhysicalDomain=network_engine_domain  SubClassName=ps_output  LeftPortType=input  RightPortType=output  PseudoPeriodic=off  Frequencies=[]  VectorFormat=1-D array  Unit=1  AffineConversion=off
  + : PMIOPort  Side=Left
  - : PMIOPort  Port=2  Side=Right
  I : Outport
  wires:
  PS-Simulink/I/1 -> I/1
  connections:
  -/RConn1 -- Current Sensor/RConn2
  Current Sensor/LConn1 -- +/RConn1
  Current Sensor/RConn1 -- PS-Simulink/I/LConn1
